simulink model "virtualwall"  (R2017a)
settings: Solver=FixedStepDiscrete  StartTime=0.0  StopTime=inf  RelTol=1e-3  EnableMultiTasking=on
undefined symbols (not defined in the file or in its folder): DiscIntNeverNeededParam, Down, GPTRIP1SEL, GPTRIP2SEL, PWM_Counter_Period, TZ1, TZ2, Up
libraries: c2806xlib x2, c2802xlib x2, c280xlib x2, simulink x1, dspsrcs4 x1, dspsigops x1
settings Model: ExtModeTrigDuration=10  Creator=Kalman  LastModifiedBy=ata.otaran
settings DataIOCC: LimitDataPoints=on  SaveFormat=Array
settings OptimizationCC: LifeSpan=Inf  MaxStackSize=512
settings DebuggingCC: AllowSymbolicDim=off  SFUnexpectedBacktrackingDiag=warning  SFNoUnconditionalDefaultTransitionDiag=warning  SFExecutionAtInitializationDiag=none
settings HardwareCC: ProdBitPerChar=16  ProdBitPerInt=16  ProdBitPerPointer=16  ProdBitPerSizeT=32  ProdBitPerPtrDiffT=32  ProdLargestAtomicInteger=Integer  ProdLargestAtomicFloat=None  ProdWordSize=16  ProdLongLongMode=on  ProdHWDeviceType=Texas Instruments->C2000
settings ModelReferenceCC: PropagateSignalLabelsOutOfModel=off
settings SFSimCC: MATLABDynamicMemAlloc=off
settings RTWCC: SystemTargetFile=ert.tlc  HardwareBoard=TI Piccolo F2806x  TLCOptions=-aInlineSetEventsForThisBaseRateFcn=TLC_FALSE -aSuppressMultiTaskScheduler=TLC_FALSE -aRateBasedStepFcn=1  TemplateMakefile=ert_default_tmf  Description=Embedded Coder  Toolchain=Texas Instruments Code Composer Studio v5 (C2000)
settings CodeAppCC: IgnoreCustomStorageClasses=off
settings ERTTargetCC: CodeReplacementLibrary=TI C28x  MultiwordLength=2048  ConvertIfToSwitch=off  SuppressUnreachableDefaultCases=off
settings ConfigComp: CovMetricSettings=dw  CovHtmlReporting=on  CovSaveCumulativeToWorkspaceVar=on  CovSaveSingleToWorkspaceVar=on  CovExternalEMLEnable=off

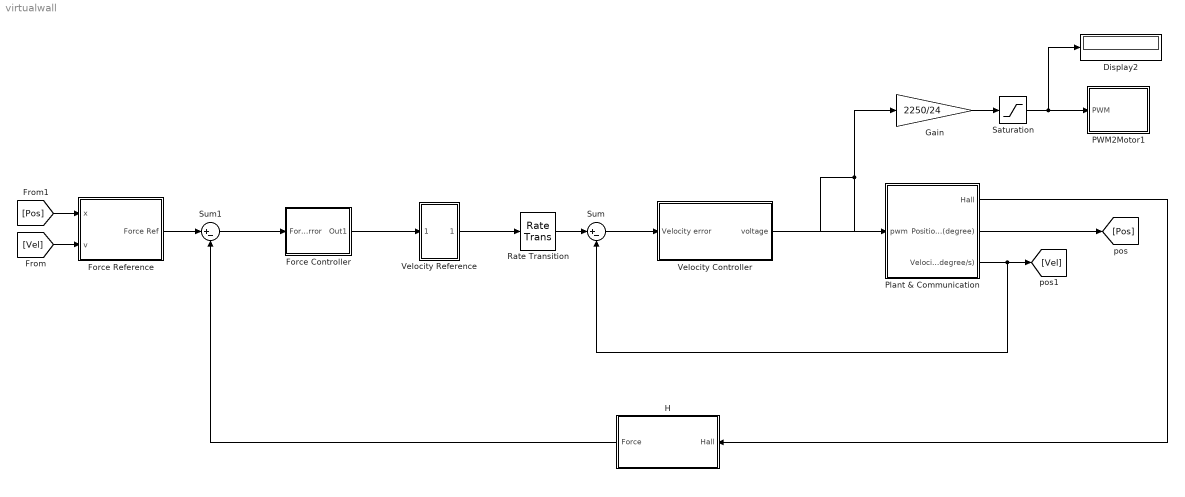
== system virtualwall ==
  Display2 : Display
  Force Controller : Subsystem
  Force Reference : Subsystem
  Gain : Gain  Gain=2250/24
  H : Subsystem
  PWM2Motor1 : Subsystem
  Plant & Communication : Subsystem
  Rate Transition : RateTransition
  Saturation : Saturate  UpperLimit=2250  LowerLimit=-2250
  Sum : Sum  Inputs=|+-
  Sum1 : Sum  Inputs=|+-
  Velocity Controller : Subsystem
  Velocity Reference : Subsystem
  wires:
  Plant & Communication/2("Position(degree) ") -> [Pos]
  Saturation/1 -> PWM2Motor1/1(PWM), Display2/1
  Plant & Communication/3(Velocity(degree/s)) -> [Vel], Sum/2
  Sum/1 -> Velocity Controller/1("Velocity error ")
  Force Reference/1(Force Ref) -> Sum1/1
  Velocity Reference/1(Out1) -> Rate Transition/1
  Velocity Controller/1(voltage) -> Gain/1, Plant & Communication/1(pwm)
  [Vel] -> Force Reference/2("v ")
  [Pos] -> Force Reference/1(x)
  Rate Transition/1 -> Sum/1
  Plant & Communication/1("Hall ") -> H/1(Hall)
  Force Controller/1(Out1) -> Velocity Reference/1(In1)
  Sum1/1 -> Force Controller/1(Force error)
  Gain/1 -> Saturation/1
  H/1(Force) -> Sum1/2

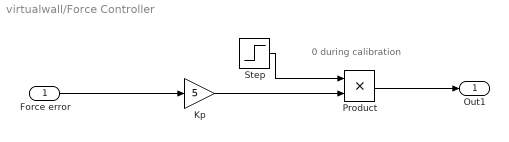
== system virtualwall/Force Controller ==
  note: 0 during calibration
  Force error : Inport
  Kp : Gain  Gain=5
  Product : Product
  Step : Step  Time=0.2
  Out1 : Outport
  wires:
  Force error/1 -> Kp/1
  Product/1 -> Out1/1
  Kp/1 -> Product/2
  Step/1 -> Product/1

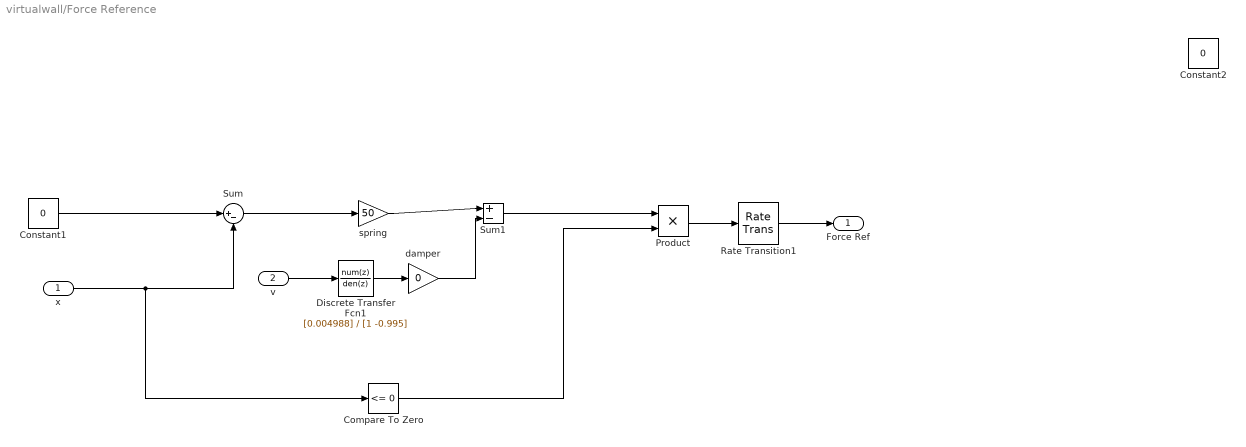
== system virtualwall/Force Reference ==
  x : Inport
  "v " : Inport  Port=2
  Compare To Zero : simulink/Logic and Bit Operations/Compare To Zero  relop=<=  OutDataTypeStr=boolean
  Constant1 : Constant  Value=0
  Constant2 : Constant  Value=0
  Discrete Transfer Fcn1 : DiscreteTransferFcn  Numerator=[0.004988]  Denominator=[1 -0.995]
  Product : Product
  Rate Transition1 : RateTransition  OutPortSampleTime=0.001
  Sum : Sum  Inputs=|+-
  Sum1 : Sum  Inputs=|+-
  damper : Gain  Gain=0
  spring : Gain  Gain=50
  Force Ref : Outport
  wires:
  Constant1/1 -> Sum/1
  Sum/1 -> spring/1
  damper/1 -> Sum1/2
  x/1 -> Compare To Zero/1, Sum/2
  Sum1/1 -> Product/1
  Compare To Zero/1 -> Product/2
  Product/1 -> Rate Transition1/1
  Rate Transition1/1 -> Force Ref/1
  "v "/1 -> Discrete Transfer Fcn1/1
  spring/1 -> Sum1/1
  Discrete Transfer Fcn1/1 -> damper/1

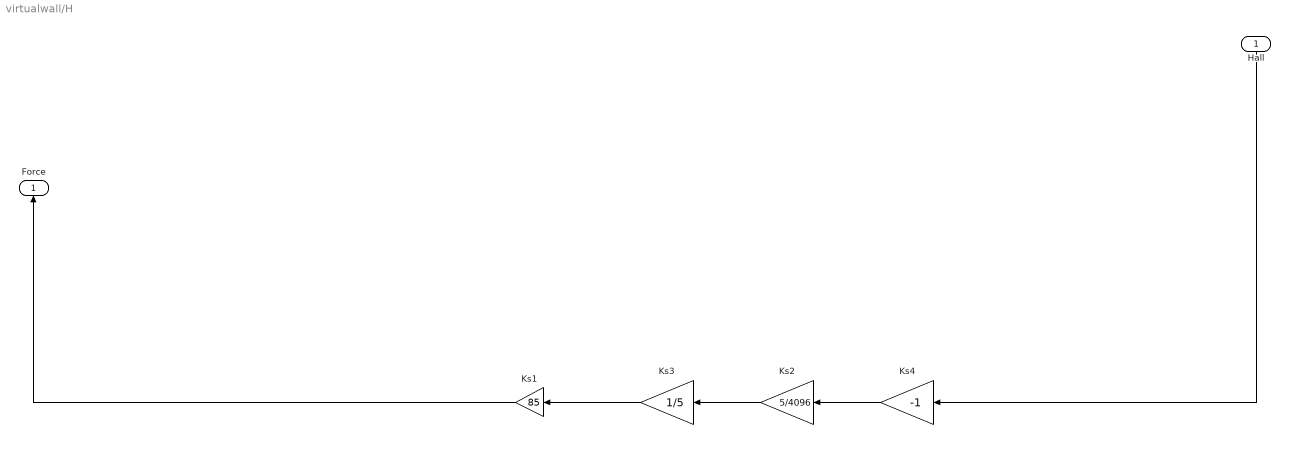
== system virtualwall/H ==
  Hall : Inport
  Ks1 : Gain  Gain=85
  Ks2 : Gain  Gain=5/4096
  Ks3 : Gain  Gain=1/5
  Ks4 : Gain  Gain=-1
  Force : Outport
  wires:
  Hall/1 -> Ks4/1
  Ks1/1 -> Force/1
  Ks4/1 -> Ks2/1
  Ks2/1 -> Ks3/1
  Ks3/1 -> Ks1/1

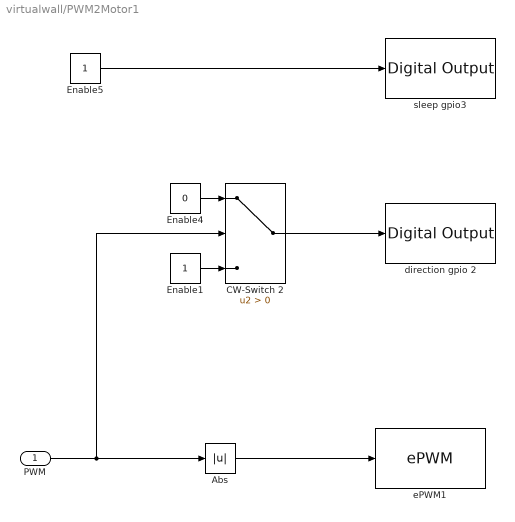
== system virtualwall/PWM2Motor1 ==
  PWM : Inport
  Abs : Abs
  CW-Switch 2 : Switch  Criteria=u2 > Threshold
  Enable1 : Constant
  Enable4 : Constant  Value=0
  Enable5 : Constant
  direction gpio 2 : c2806xlib/Digital Output  GPIO_Number=GPIO0~GPIO7  GPIO_Bit0=off  GPIO_BIT0_Toggle=off  GPIO_Bit1=off  GPIO_BIT1_Toggle=off  GPIO_Bit2=on  GPIO_BIT2_Toggle=off  GPIO_Bit3=off  GPIO_BIT3_Toggle=off  GPIO_Bit4=off  GPIO_BIT4_Toggle=off  GPIO_Bit5=off  GPIO_BIT5_Toggle=off  GPIO_Bit6=off  GPIO_BIT6_Toggle=off  GPIO_Bit7=off  GPIO_BIT7_Toggle=off
      settings: SourceProductName=Embedded Coder Support Package for Texas Instruments C2000 Processors  SourceProductBaseCode=TIC2000
  ePWM1 : c2802xlib/ePWM  useModule=ePWM1  ePWMxLINKTBPRD=Not Linked  periodUnits=Clock cycles  timerSource=Specify via dialog  timerPeriod_clk=PWM_Counter_Period+1  timerPeriod_sec=0.0001  tbshadow=Counter equals to zero  countingMode=Up-Down  phaseActiveEnable=Disable  phaseDirection=Count down after sync  phaseActive=0  synchronizationEnable=off  dcaevt1Sync=off  dcbevt1Sync=off  synchronizationOption=Disable  clockPrescale=1  HSclockPrescale=1  enswap=off  ePWMxAStatus=on  ePWMxAactionLogic1=Do nothing  ePWMxAactionLogic2=Do nothing  ePWMxAactionLogic3=Clear  ePWMxAactionLogic4=Set  ePWMxAactionLogic5=Do nothing  ePWMxAactionLogic6=Do nothing  ePWMxALoadMode=Load on counter equals to zero (CTR=Zero)  ePWMxACSFenable=off  ePWMxACSFvalue=Forcing disable  ePWMxASFreload=Zero  ePWMxBStatus=off  ePWMxBactionLogic1=Set  ePWMxBactionLogic2=Clear  ePWMxBactionLogic3=Do nothing  ePWMxBactionLogic4=Do nothing  ePWMxBactionLogic5=Clear  ePWMxBactionLogic6=Set  ePWMxBLoadMode=Load on counter equals to zero (CTR=Zero)  ePWMxBCSFenable=off  ePWMxBCSFvalue=Forcing disable  ePWMxBSFreload=Zero  ePWNxBOutWay=off  ePWMxLINKCMPA=Not Linked  CMPAUnits=Clock cycles  CMPASource=Input port  CMPAValue_per=50  CMPAValue_clk=PWM_Counter_Period/2+1  enCMPAshadow=Counter equals to zero  ePWMxLINKCMPB=Not Linked  CMPBUnits=Clock cycles  CMPBSource=Specify via dialog  CMPBValue_per=50  CMPBValue_clk=PWM_Counter_Period/2+1  enCMPBshadow=Counter equals to zero  ePWMxLINKCMPC=Not Linked  CMPCUnits=Clock cycles  CMPCSource=Specify via dialog  CMPCValue_per=50  CMPCValue_clk=32000  enCMPCshadow=Counter equals to zero  ePWMxLINKCMPD=Not Linked  CMPDUnits=Clock cycles  CMPDSource=Specify via dialog  CMPDValue_per=50  CMPDValue_clk=32000  enCMPDshadow=Counter equals to zero  enableDBePWMxA=off  enableDBePWMxB=off  enhalfcycle=off  DBpolarity=Active high (AH)  DBedgeDelay=Positive  DBSource_ePWMxA=ePWMxA  DBSource_ePWMxB=ePWMxA  DBperiodSource=Specify via dialog  REDperiod=0  FEDperiod=0  adcstartModuleA=off  adcrequestEventA=First event  adcstartEventA=Digital Compare Module A Event 1 start of conversion (DCAEVT1.soc)  adcstartEventA_type2=Digital Compare Module A Event 1 start of conversion (DCAEVT1.soc)  adcstartModuleB=off  adcrequestEventB=First event  adcstartEventB=Counter equals to zero (CTR=Zero)  adcstartEventB_type2=Counter equals to zero (CTR=Zero)  intEn=off  intPrd=First event  intSel=Counter equals to zero (CTR=Zero)  intSel_type2=Counter equals to zero (CTR=Zero)  hrpe=off  enHRPWM=off  HRPWM_LoadMode=Counter equals to period (CTR=PRD)  HRPWM_CTLMode=Duty or Period control mode  HRPWM_EDGMode=Both edge  hrpeb=off  enHRPWMB=off  HRPWM_LoadModeB=Counter equals to zero (CTR=ZERO)  HRPWM_CTLModeB=Duty or Period control mode  HRPWM_EDGModeB=Both edge  enSFO=on  enautoconv=on  chopperEnable=off  chopperFrequency=1  chopperFirstwidth=1  chopperDuty=12.5%  tripZonesource=Specify via dialog  tzselOSHT1=off  tzselOSHT2=off  tzselOSHT3=off  tzselOSHDCAEV1=off  tzselOSHDCBEV1=off  tzselCBC1=off  tzselCBC2=off  tzselCBC3=off  tzselCBCDCAEV2=off  tzselCBCDCBEV2=off  tzselOSHT4=off  tzselOSHT5=off  tzselOSHT6=off  tzselCBC4=off  tzselCBC5=off  tzselCBC6=off  enTzOstIntr=off  enTzCbcIntr=off  enTzDCAEVT1Intr=off  enTzDCAEVT2Intr=off  enTzDCBEVT1Intr=off  enTzDCBEVT2Intr=off  ePWMxAforced=No action  ePWMxBforced=No action  DCAEVT1forced=No action  DCBEVT1forced=No action  DCAEVT2forced=No action  DCBEVT2forced=No action  dcah=Trip Zone 1 input (TZ1)  dcal=Trip Zone 2 input (TZ2)  dcbh=Trip Zone 1 input (TZ1)  dcbl=Trip Zone 2 input (TZ2)  dcah_type2=GPTRIP1SEL/(TZ1)  dcal_type2=GPTRIP2SEL/(TZ2)  dcbh_type2=GPTRIP1SEL/(TZ1)  dcbl_type2=GPTRIP2SEL/(TZ2)  gendcaevt1=Event disabled  gendcaevt2=Event disabled  gendcbevt1=Event disabled  gendcbevt2=Event disabled  dcaevt1src=DCAEVT1 with sync  dcaevt2src=DCAEVT2 with sync  dcbevt1src=DCBEVT1 with sync  dcbevt2src=DCBEVT2 with sync  pulsesel=Counter equals to zero (CTR=Zero)  blankinv=off  blankoffset=0  blankwidth=0  evsrcsel=Filtered version of DCAEVT1 (DCAEVT1FILT)  encape=off  PwmType=C2000
      settings: SourceProductName=Embedded Coder Support Package for Texas Instruments C2000 Processors
  sleep gpio3 : c2806xlib/Digital Output  GPIO_Number=GPIO0~GPIO7  GPIO_Bit0=off  GPIO_BIT0_Toggle=off  GPIO_Bit1=off  GPIO_BIT1_Toggle=off  GPIO_Bit2=off  GPIO_BIT2_Toggle=off  GPIO_Bit3=on  GPIO_BIT3_Toggle=off  GPIO_Bit4=off  GPIO_BIT4_Toggle=off  GPIO_Bit5=off  GPIO_BIT5_Toggle=off  GPIO_Bit6=off  GPIO_BIT6_Toggle=off  GPIO_Bit7=off  GPIO_BIT7_Toggle=off
      settings: SourceProductName=Embedded Coder Support Package for Texas Instruments C2000 Processors  SourceProductBaseCode=TIC2000
  wires:
  PWM/1 -> Abs/1, CW-Switch 2/2
  Enable1/1 -> CW-Switch 2/3
  Enable4/1 -> CW-Switch 2/1
  Enable5/1 -> sleep gpio3/1
  CW-Switch 2/1 -> direction gpio 2/1
  Abs/1 -> ePWM1/1

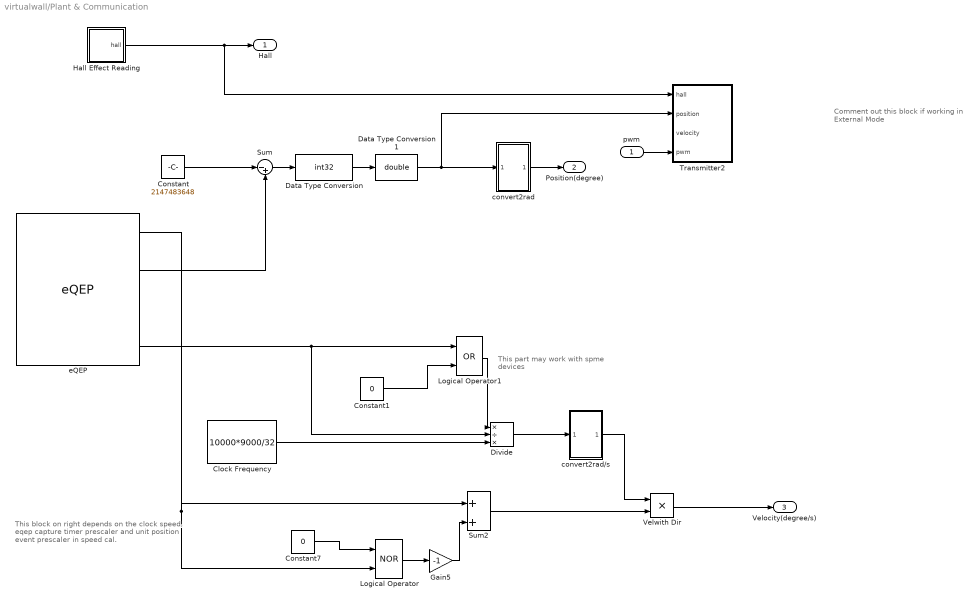
== system virtualwall/Plant & Communication ==
  note: This part may work with
      | spme devices
  note: Comment out this block if
      | working in External Mode
  note: This block on right depends on the clock speed, eqep capture timer prescaler and
      | unit position event prescaler in speed cal.
  pwm : Inport
  Clock Frequency : Constant  Value=10000*9000/32
  Constant : Constant  Value=2147483648  OutDataTypeStr=uint32
  Constant1 : Constant  Value=0
  Constant7 : Constant  Value=0
  Data Type Conversion : DataTypeConversion  OutDataTypeStr=int32
  Data Type Conversion1 : DataTypeConversion  OutDataTypeStr=double
  Divide : Product  Inputs=*/*
  Gain5 : Gain  Gain=-1
  Hall Effect Reading : Subsystem
  Logical Operator : Logic  Operator=NOR  AllPortsSameDT=off  OutDataTypeStr=boolean
  Logical Operator1 : Logic  Operator=OR  AllPortsSameDT=off  OutDataTypeStr=boolean
  Sum : Sum  Inputs=|-+
  Sum2 : Sum  Inputs=|++
  Transmitter2 : Subsystem
  "Velwith Dir " : Product
  convert2rad : Subsystem
  convert2rad/s : Subsystem
  eQEP : c280xlib/eQEP  useModule=eQEP1  pcInputmode=Quadrature-count  externalClockrate=2x resolution: Count the rising/falling edge  swapPolarityselection=Clockwise  qdfOutputport=on  qapPolarityselection=off  qbpPolarityselection=off  qipPolarityselection=off  qspPolarityselection=off  igatePolarityselection=off  sampleTime=0.0001  pcOutputport=on  pcMaximumvalue=4294967295  indexInitializationcheck=off  indexInitializationevent=Rising edge  strobeInitializationcheck=off  strobeInitializationevent=Rising edge  softwareInitializationcheck=on  softwareInitializationsource=Set to init value at start up  softwareInitializationmode=on  pcInitialvalue=2147483648  pcResetmode=Reset on an index event  ieloutputport=off  indexEventlatch=Rising edge  seloutputport=off  strobeEventlatch=Rising edge  pcefOutputport=off  enableEqepcapture=on  qctmrOutputport=on  qcprdOutputport=on  captureTimerprescaler=128  upEventprescaler=4  overflowErrorflag=off  directionErrorflag=off  captureTimerposition=On position counter read  unitTimerperiod=1000000000  captureTimerlatch=off  capturePeriodlatch=off  positionCounterlatch=off  soenPolarityselection=off  spselPolarityselection=Index pin is used for sync output  compareValuesource=Specify via dialog  shadowMode=Load on QPOSCNT=0  compareValue=4294967295  syncOutputwidth=1  polaritySyncoutput=Active high  watchdogEnable=off  watchdogTimer=65535  outport1Datatype=auto  outport2Datatype=uint32  outport3Datatype=auto  outport4Datatype=auto  outport5Datatype=auto  outport6Datatype=auto  outport7Datatype=auto  outport8Datatype=auto  outport9Datatype=auto  outport10Datatype=auto  outport11Datatype=auto  outport12Datatype=auto  eqepinterrupt_pce=off  eqepinterrupt_qpe=off  eqepinterrupt_qdc=off  eqepinterrupt_wto=off  eqepinterrupt_pcu=off  eqepinterrupt_pco=off  eqepinterrupt_pcr=off  eqepinterrupt_pcm=off  eqepinterrupt_sel=off  eqepinterrupt_iel=off  eqepinterrupt_uto=off  pheOutputport=off  watchdogOutputport=off  outport13Datatype=auto  outport14Datatype=auto
      settings: SourceProductName=Embedded Coder Support Package for Texas Instruments C2000 Processors  SourceProductBaseCode=TIC2000
  "Hall " : Outport
  "Position(degree) " : Outport  Port=2
  Velocity(degree/s) : Outport  Port=3
  wires:
  convert2rad/s/1(Out1) -> "Velwith Dir "/1
  Hall Effect Reading/1(hall) -> Transmitter2/1(hall), "Hall "/1
  Logical Operator1/1 -> Divide/1
  Clock Frequency/1 -> Divide/3
  Constant1/1 -> Logical Operator1/2
  Sum2/1 -> "Velwith Dir "/2
  Constant7/1 -> Logical Operator/1
  Logical Operator/1 -> Gain5/1
  Divide/1 -> convert2rad/s/1(In1)
  Gain5/1 -> Sum2/2
  eQEP/1 -> Logical Operator/2, Sum2/1
  eQEP/2 -> Sum/2
  Constant/1 -> Sum/1
  eQEP/4 -> Logical Operator1/1, Divide/2
  Data Type Conversion/1 -> Data Type Conversion1/1
  convert2rad/1(Out1) -> "Position(degree) "/1
  Sum/1 -> Data Type Conversion/1
  Data Type Conversion1/1 -> Transmitter2/2(position), convert2rad/1(In1)
  pwm/1 -> Transmitter2/4(pwm)
  "Velwith Dir "/1 -> Velocity(degree/s)/1

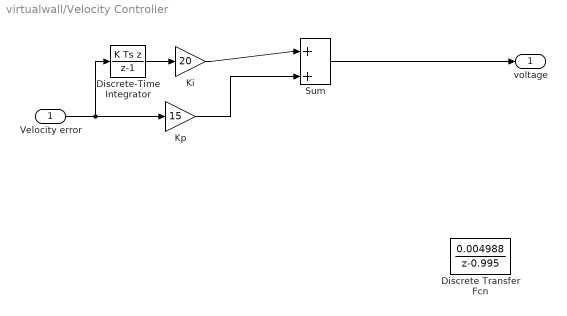
== system virtualwall/Velocity Controller ==
  "Velocity error " : Inport
  Discrete Transfer Fcn : DiscreteTransferFcn  Numerator=[0.004988]  Denominator=[1 -0.995]
  Discrete-Time Integrator : DiscreteIntegrator  IntegratorMethod=Integration: Backward Euler  InitialConditionSetting=State (most efficient)  SampleTime=-1  ICPrevOutput=DiscIntNeverNeededParam  ICPrevScaledInput=DiscIntNeverNeededParam
  Ki : Gain  Gain=20
  Kp : Gain  Gain=15
  Sum : Sum  Inputs=|++
  voltage : Outport
  wires:
  "Velocity error "/1 -> Kp/1, Discrete-Time Integrator/1
  Kp/1 -> Sum/2
  Ki/1 -> Sum/1
  Discrete-Time Integrator/1 -> Ki/1
  Sum/1 -> voltage/1

== system virtualwall/Velocity Reference ==
  In1 : Inport
  Out1 : Outport
  wires:
  In1/1 -> Out1/1

== system virtualwall/Plant & Communication/Hall Effect Reading ==
  ADC2 : c2802xlib/ADC  ADCModule=1  samplingMode=Single sample mode  ADCResolution=12-bit (Single-ended input)  useSOC1=SOC1  useSOC2=SOC0_SOC1  SOCAcquisitionWindow=7  SOCTriggerSource=Software  SOCInterruptTrigger=No ADCINT  Ts=-1  dType=int32  postInterrupt=off  interruptSel=ADCINT1  ADCINTContinuous=off  endma=off  chdma=1  blkParamProc=C2000  conv1=ADCINA7  conv2=ADCINA7 and ADCINB7  conv1_Type4=ADCIN0  conv2_Type4=ADCIN0 and ADCIN1
      settings: SourceProductName=Embedded Coder Support Package for Texas Instruments C2000 Processors
  Automatic Calibration : Subsystem
  Signal Processing : Subsystem
  hall : Outport
  wires:
  ADC2/1 -> Automatic Calibration/1(raw)
  Automatic Calibration/1(calibrated) -> Signal Processing/1(raw)
  Signal Processing/1(filtered) -> hall/1

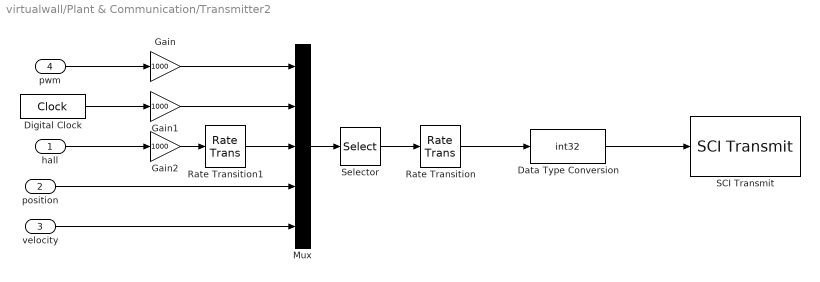
== system virtualwall/Plant & Communication/Transmitter2 ==
  hall : Inport
  position : Inport  Port=2
  velocity : Inport  Port=3
  pwm : Inport  Port=4
  Data Type Conversion : DataTypeConversion  OutDataTypeStr=int32  ConvertRealWorld=Stored Integer (SI)
  Digital Clock : DigitalClock  SampleTime=0.0001
  Gain : Gain  Gain=1000
  Gain1 : Gain  Gain=1000
  Gain2 : Gain  Gain=1000
  Mux : Mux  Inputs=5
  Rate Transition : RateTransition  Integrity=off  OutPortSampleTime=0.03
  Rate Transition1 : RateTransition  Integrity=off  OutPortSampleTime=0.0001
  SCI Transmit : c280xlib/SCI Transmit  sciModule=A  dataHead='S'  dataTail='E'  postInterrupt=on  numFifo=3
      settings: SourceProductName=Embedded Coder Support Package for Texas Instruments C2000 Processors
  Selector : Selector  InputPortWidth=5  IndexOptions=Index vector (dialog)  Indices=[3 4]  OutputSizes=1
  wires:
  Rate Transition/1 -> Data Type Conversion/1
  Data Type Conversion/1 -> SCI Transmit/1
  velocity/1 -> Mux/5
  Digital Clock/1 -> Gain1/1
  Gain/1 -> Mux/1
  pwm/1 -> Gain/1
  hall/1 -> Gain2/1
  Mux/1 -> Selector/1
  Gain1/1 -> Mux/2
  Gain2/1 -> Rate Transition1/1
  Selector/1 -> Rate Transition/1
  position/1 -> Mux/4
  Rate Transition1/1 -> Mux/3

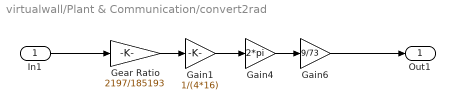
== system virtualwall/Plant & Communication/convert2rad ==
  In1 : Inport
  Gain1 : Gain  Gain=1/(4*16)
  Gain4 : Gain  Gain=2*pi
  Gain6 : Gain  Gain=9/73
  Gear Ratio : Gain  Gain=2197/185193
  Out1 : Outport
  wires:
  Gain1/1 -> Gain4/1
  Gear Ratio/1 -> Gain1/1
  Gain4/1 -> Gain6/1
  In1/1 -> Gear Ratio/1
  Gain6/1 -> Out1/1

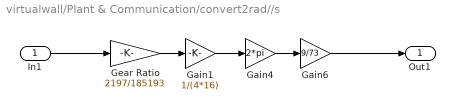
== system virtualwall/Plant & Communication/convert2rad//s ==
  In1 : Inport
  Gain1 : Gain  Gain=1/(4*16)
  Gain4 : Gain  Gain=2*pi
  Gain6 : Gain  Gain=9/73
  Gear Ratio : Gain  Gain=2197/185193
  Out1 : Outport
  wires:
  Gain6/1 -> Out1/1
  In1/1 -> Gear Ratio/1
  Gain4/1 -> Gain6/1
  Gear Ratio/1 -> Gain1/1
  Gain1/1 -> Gain4/1

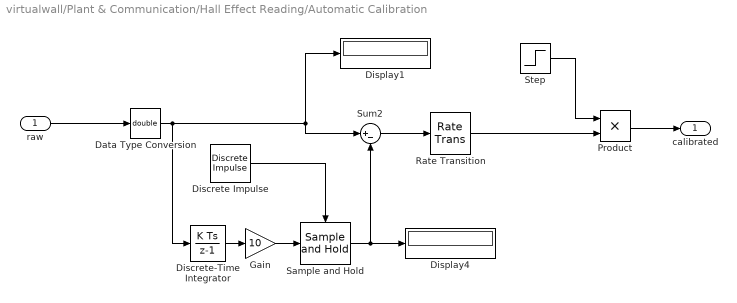
== system virtualwall/Plant & Communication/Hall Effect Reading/Automatic Calibration ==
  raw : Inport
  Data Type Conversion : DataTypeConversion  OutDataTypeStr=double
  Discrete Impulse : dspsrcs4/Discrete  Impulse  Delay=1000  SampleTime=-1  FrameSample=1  OutputFrames=off  dataType=double  isSigned=on  wordLen=16  udDataType=sfix(16)  fracBitsMode=Best precision  numFracBits=15  OutDataTypeStr=double  LastOutDataTypeStr=double
  Discrete-Time Integrator : DiscreteIntegrator  InitialConditionSetting=State (most efficient)  SampleTime=1e-4  ICPrevOutput=DiscIntNeverNeededParam  ICPrevScaledInput=DiscIntNeverNeededParam
  Display1 : Display
  Display4 : Display
  Gain : Gain  Gain=10
  Product : Product
  Rate Transition : RateTransition
  Sample and Hold : dspsigops/Sample and Hold  trig=Rising edge  initCond=0  latchinput=off
  Step : Step  Time=0.1  SampleTime=1e-4
  Sum2 : Sum  Inputs=|+-
  calibrated : Outport
  wires:
  raw/1 -> Data Type Conversion/1
  Discrete Impulse/1 -> Sample and Hold/Trigger
  Data Type Conversion/1 -> Discrete-Time Integrator/1, Sum2/1, Display1/1
  Sample and Hold/1 -> Display4/1, Sum2/2
  Discrete-Time Integrator/1 -> Gain/1
  Gain/1 -> Sample and Hold/1
  Sum2/1 -> Rate Transition/1
  Rate Transition/1 -> Product/2
  Step/1 -> Product/1
  Product/1 -> calibrated/1

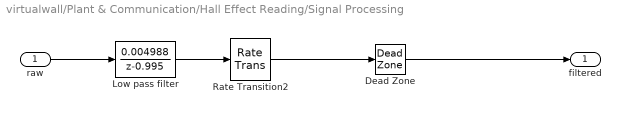
== system virtualwall/Plant & Communication/Hall Effect Reading/Signal Processing ==
  raw : Inport
  Dead Zone : DeadZone  LowerValue=-2  UpperValue=2  SaturateOnIntegerOverflow=on
  Low pass filter : DiscreteTransferFcn  Numerator=[0.004988]  Denominator=[1 -0.995]
  Rate Transition2 : RateTransition  OutPortSampleTime=0.001
  filtered : Outport
  wires:
  raw/1 -> Low pass filter/1
  Rate Transition2/1 -> Dead Zone/1
  Low pass filter/1 -> Rate Transition2/1
  Dead Zone/1 -> filtered/1
